simulink model "lab2_part3_model"  (R2025a)
settings: Solver=ode45  StartTime=0.0  StopTime=3.0  MaxStep=0.001  RelTol=1e-3
model workspace (MAT data in the model file):
  a = 10
  zeta = 10
values from neighbouring files (symbols this model uses):
  a1 = -30    [lab2_part2.m]    (also in lab2_part3.m = -0.5)
  zeta1 = 0.6    [lab2_part2.m]    (also in lab2_part3.m)
settings Model: Creator=marksorial  LastModifiedBy=marksorial

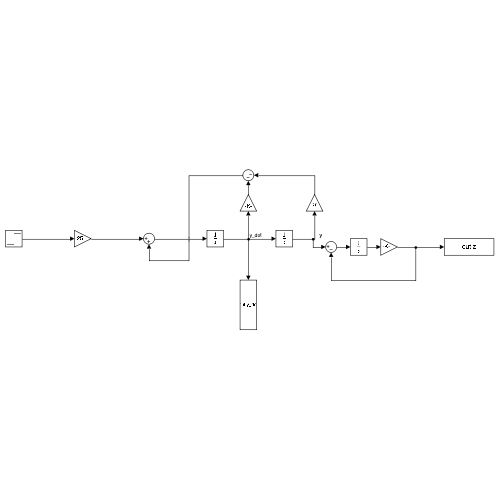
[thumbnail: Simulink's stored preview of the top-level diagram]
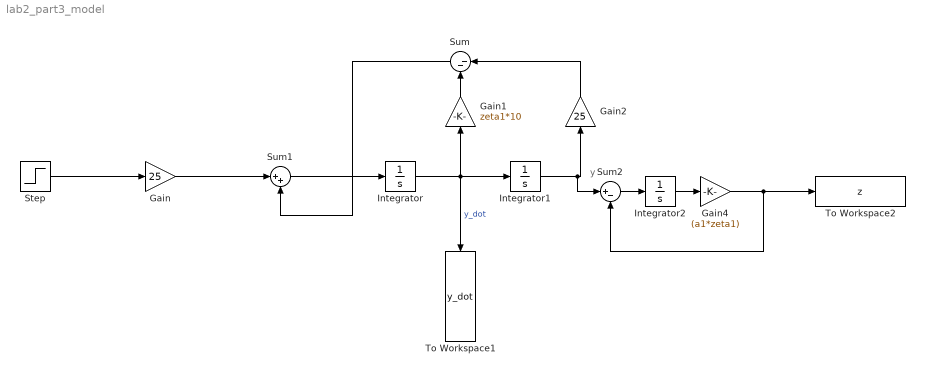
== system lab2_part3_model ==
  note: y
  Gain : Gain  Gain=25
  Gain1 : Gain  Gain=zeta1*10
  Gain2 : Gain  Gain=25
  Gain4 : Gain  Gain=(a1*zeta1)
  Integrator : Integrator
  Integrator1 : Integrator
  Integrator2 : Integrator
  Step : Step  Time=0  SampleTime=0
  Sum : Sum  Inputs=|--
  Sum1 : Sum  Inputs=|++
  Sum2 : Sum  Inputs=|+-
  To Workspace1 : ToWorkspace  VariableName=y_dot  SampleTime=-1
      settings: Save2DSignal=2-D array (concatenate along first dimension)
  To Workspace2 : ToWorkspace  VariableName=z  SampleTime=-1
      settings: Save2DSignal=2-D array (concatenate along first dimension)
  wires:
  Integrator/1 -> To Workspace1/1, Gain1/1, Integrator1/1  "y_dot"
  Step/1 -> Gain/1
  Gain1/1 -> Sum/2
  Gain2/1 -> Sum/1
  Gain/1 -> Sum1/1
  Sum/1 -> Sum1/2
  Sum1/1 -> Integrator/1
  Integrator1/1 -> Sum2/1, Gain2/1
  Integrator2/1 -> Gain4/1
  Sum2/1 -> Integrator2/1
  Gain4/1 -> Sum2/2, To Workspace2/1
